simulink model "motor_control"  (Simulink 7.9)
settings: Solver=ode45  StartTime=0.0  StopTime=1  RelTol=1e-3
libraries: powerlib x10
settings Model: Creator=Dmitriy  LastModifiedBy=Dmitriy
settings GRTTargetCC: CombineOutputUpdateFcns=off  GRTInterface=on

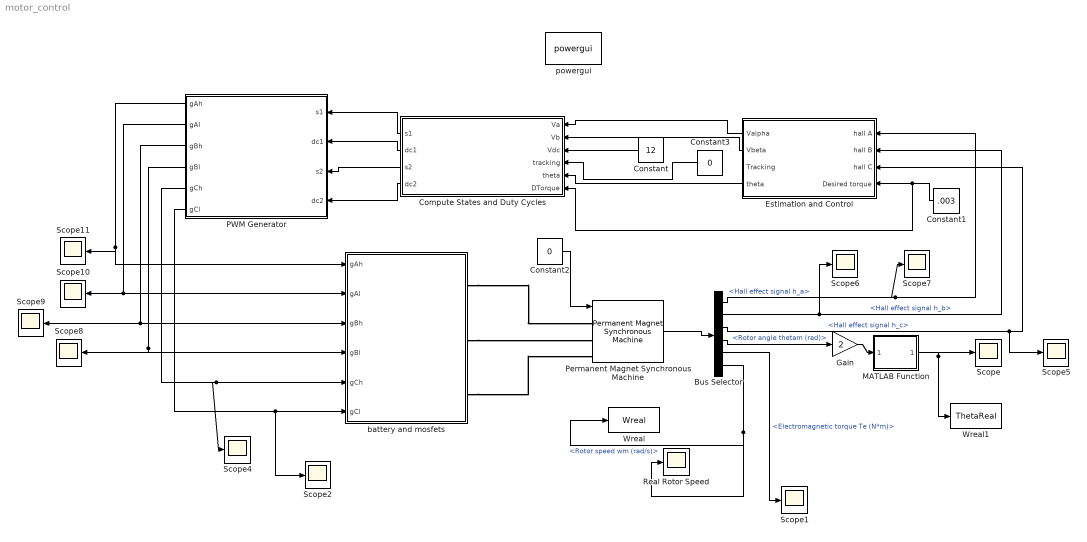
== system motor_control ==
  Bus Selector : BusSelector  OutputSignals=Hall effect signal h_a,Hall effect signal h_b,Hall effect signal h_c,Rotor angle thetam (rad),Electromagnetic torque Te (N*m),Rotor speed wm (rad/s)
  Compute States and Duty Cycles : MATLAB Function  TreatAsAtomicUnit=on  SystemSampleTime=.001
  Constant : Constant  Value=12
  Constant1 : Constant  Value=.003
  Constant2 : Constant  Value=0
  Constant3 : Constant  Value=0
  Estimation and Control : Subsystem  SystemSampleTime=.001
  Gain : Gain  Gain=2
  MATLAB Function : MATLAB Function  TreatAsAtomicUnit=on
  PWM Generator : MATLAB Function  TreatAsAtomicUnit=on  SystemSampleTime=10^-6
  Permanent Magnet Synchronous Machine : powerlib/Machines/Permanent Magnet Synchronous Machine  NbPhases=3  FluxDistribution=Sinusoidal  RotorType=Round  MechanicalLoad=Torque Tm  PresetModel=No  ShowDetailedParameters=on  Resistance=28.2  Inductance=8.5e-3  dqInductances=[0.006365 0.006365]  La=1940*10^-6  MachineConstant=Torque Constant (N.m / A_peak)  Flux=0.0060333  VoltageCst=2.1887  TorqueCst=0.0181  Flat=120  Mechanical=[0.0001 5.396e-005 2 0]  PolePairs=2  InitialConditions=[0,1, 0,0]  InitialConditions5ph=[0 0 0 0 0 0]  TsPowergui=0  TsBlock=-1  RefAngle=Aligned with phase A axis (original Park)
  Real Rotor Speed : Scope
      settings: SaveName=ScopeData18
  Scope{,1..2,4..11} (11 alike) : Scope
      Scope settings: YMin=0.2591  YMax=0.2614
      Scope10 settings: SaveName=ScopeData10
      Scope11 settings: SaveName=ScopeData11
      Scope2 settings: YMin=0.95  YMax=1.05  SaveName=ScopeData2
      Scope4 settings: YMin=0.95  YMax=1.05  SaveName=ScopeData4
      Scope5 settings: SaveName=ScopeData5
      Scope6 settings: SaveName=ScopeData6
      Scope7 settings: SaveName=ScopeData7
      Scope8 settings: SaveName=ScopeData8
      Scope9 settings: SaveName=ScopeData9
  Wreal : ToWorkspace  VariableName=Wreal  SampleTime=-1  SaveFormat=Timeseries
  Wreal1 : ToWorkspace  VariableName=ThetaReal  SampleTime=-1  SaveFormat=Timeseries
  battery and mosfets : Subsystem
  powergui : powerlib/powergui  Priority=1  SimulationMode=Continuous  SolverType=Tustin  SampleTime=50e-6  frequency=60  SPID=off  DisableSnubberDevices=off  DisableRonSwitches=off  DisableVfSwitches=off  SwTol=0  Interpol=off  DisplayEquations=off  FunctionMessages=off  frequencyindice=0  Pbase=100e6  ErrMax=1e-4  Iterations=50  UnitsV=kV  UnitsW=MW  echomessages=off  HookPort=off  EnableUseOfTLC=off  x0status=blocks  RestoreLinks=warning  ResistiveCurrentMeasurement=off  Ylog=off  Xlog=on  ShowGrid=off  save=off  variable=ZData  ZoomFFT=off  StartTime=0.0  cycles=1  DisplayStyle=1  FreqAxis=off  MaxFrequency=1000  frequencyindicesteady=1  display=off  methode=off
  wires:
  Permanent Magnet Synchronous Machine/1 -> Bus Selector/1
  Bus Selector/1 -> Estimation and Control/1(hall A), Scope7/1  "<Hall effect signal h_a>"
  Bus Selector/3 -> Estimation and Control/3(hall C), Scope5/1  "<Hall effect signal h_c>"
  Bus Selector/4 -> Gain/1  "<Rotor angle thetam (rad)>"
  Bus Selector/5 -> Scope1/1  "<Electromagnetic torque Te (N*m)>"
  Bus Selector/2 -> Estimation and Control/2(hall B), Scope6/1  "<Hall effect signal h_b>"
  Estimation and Control/1(Valpha) -> Compute States and Duty Cycles/1(Va)
  Compute States and Duty Cycles/1(s1) -> PWM Generator/1(s1)
  Compute States and Duty Cycles/2(dc1) -> PWM Generator/2(dc1)
  Compute States and Duty Cycles/3(s2) -> PWM Generator/3(s2)
  Compute States and Duty Cycles/4(dc2) -> PWM Generator/4(dc2)
  PWM Generator/6(gCl) -> battery and mosfets/6(gCl), Scope2/1
  PWM Generator/5(gCh) -> battery and mosfets/5(gCh), Scope4/1
  PWM Generator/4(gBl) -> battery and mosfets/4(gBl), Scope8/1
  PWM Generator/3(gBh) -> battery and mosfets/3(gBh), Scope9/1
  PWM Generator/2(gAl) -> battery and mosfets/2(gAl), Scope10/1
  PWM Generator/1(gAh) -> battery and mosfets/1(gAh), Scope11/1
  Constant/1 -> Compute States and Duty Cycles/3(Vdc)
  Constant1/1 -> Estimation and Control/4(Desired torque), Compute States and Duty Cycles/6(DTorque)
  Estimation and Control/2(Vbeta) -> Compute States and Duty Cycles/2(Vb)
  Bus Selector/6 -> Real Rotor Speed/1, Wreal/1  "<Rotor speed wm (rad/s)>"
  MATLAB Function/1(lambda1) -> Wreal1/1, Scope/1
  Gain/1 -> MATLAB Function/1(lambda)
  Constant2/1 -> Permanent Magnet Synchronous Machine/1
  Estimation and Control/4(theta) -> Compute States and Duty Cycles/5(theta)
  Constant3/1 -> Compute States and Duty Cycles/4(tracking)
  connections:
  battery and mosfets/RConn1 -- Permanent Magnet Synchronous Machine/LConn1
  battery and mosfets/RConn2 -- Permanent Magnet Synchronous Machine/LConn2
  battery and mosfets/RConn3 -- Permanent Magnet Synchronous Machine/LConn3

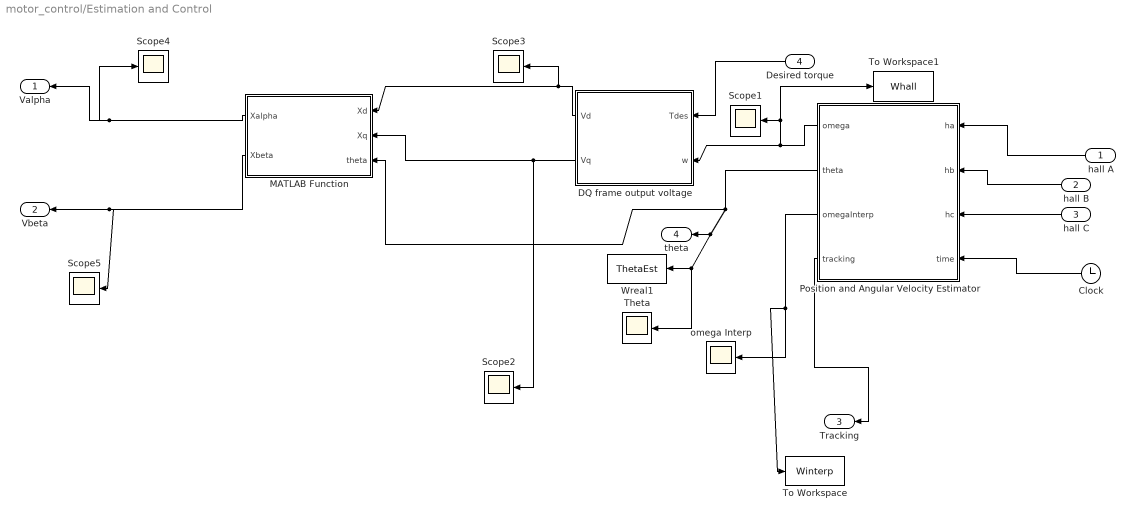
== system motor_control/Estimation and Control ==
  hall A : Inport
  hall B : Inport  Port=2
  hall C : Inport  Port=3
  Desired torque : Inport  Port=4
  Clock : Clock
  DQ frame output voltage : MATLAB Function  TreatAsAtomicUnit=on  SystemSampleTime=.0001
  MATLAB Function : MATLAB Function  TreatAsAtomicUnit=on
  Position and Angular Velocity Estimator : MATLAB Function  TreatAsAtomicUnit=on  SystemSampleTime=.0001
  Scope{1..5} (5 alike) : Scope
      Scope1 settings: SaveName=ScopeData13
      Scope2 settings: SaveName=ScopeData14
      Scope3 settings: SaveName=ScopeData15
      Scope4 settings: SaveName=ScopeData16
      Scope5 settings: SaveName=ScopeData17
  Theta : Scope
      settings: YMin=0  YMax=3.25  SaveName=ScopeData12
  To Workspace : ToWorkspace  VariableName=Winterp  SampleTime=-1  SaveFormat=Timeseries
  To Workspace1 : ToWorkspace  VariableName=Whall  SampleTime=-1  SaveFormat=Timeseries
  Wreal1 : ToWorkspace  VariableName=ThetaEst  SampleTime=-1  SaveFormat=Timeseries
  omega Interp : Scope
      settings: YMin=0  YMax=3.25  SaveName=ScopeData19
  Valpha : Outport
  Vbeta : Outport  Port=2
  Tracking : Outport  Port=3
  theta : Outport  Port=4
  wires:
  Position and Angular Velocity Estimator/1(omega) -> DQ frame output voltage/2(w), Scope1/1, To Workspace1/1
  Desired torque/1 -> DQ frame output voltage/1(Tdes)
  hall A/1 -> Position and Angular Velocity Estimator/1(ha)
  hall B/1 -> Position and Angular Velocity Estimator/2(hb)
  hall C/1 -> Position and Angular Velocity Estimator/3(hc)
  Position and Angular Velocity Estimator/2(theta) -> MATLAB Function/3(theta), Theta/1, Wreal1/1, theta/1
  DQ frame output voltage/2(Vq) -> Scope2/1, MATLAB Function/2(Xq)
  DQ frame output voltage/1(Vd) -> Scope3/1, MATLAB Function/1(Xd)
  MATLAB Function/1(Xalpha) -> Valpha/1, Scope4/1
  MATLAB Function/2(Xbeta) -> Vbeta/1, Scope5/1
  Position and Angular Velocity Estimator/3(omegaInterp) -> omega Interp/1, To Workspace/1
  Clock/1 -> Position and Angular Velocity Estimator/4(time)
  Position and Angular Velocity Estimator/4(tracking) -> Tracking/1

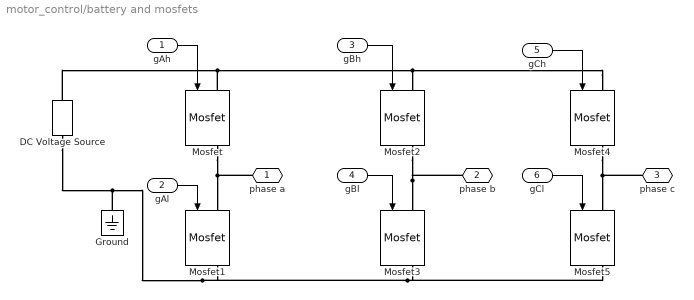
== system motor_control/battery and mosfets ==
  gAh : Inport
  gAl : Inport  Port=2
  gBh : Inport  Port=3
  gBl : Inport  Port=4
  gCh : Inport  Port=5
  gCl : Inport  Port=6
  DC Voltage Source : powerlib/Electrical Sources/DC Voltage Source  Amplitude=12  Measurements=None
  Ground : powerlib/Elements/Ground  LConnTagsString=a
  Mosfet{,1..5} (6 alike) : powerlib/Power Electronics/Mosfet  Ron=0.1  Lon=0  Rd=0.01  Vfd=0  IC=0  Rs=1e5  Cs=inf  Measurements=on
  phase a : PMIOPort  Port=1  Side=Right
  phase b : PMIOPort  Port=2  Side=Right
  phase c : PMIOPort  Port=3  Side=Right
  wires:
  gCl/1 -> Mosfet5/1
  gCh/1 -> Mosfet4/1
  gBh/1 -> Mosfet2/1
  gBl/1 -> Mosfet3/1
  gAl/1 -> Mosfet1/1
  gAh/1 -> Mosfet/1
  connections:
  Mosfet/RConn1 -- Mosfet1/LConn1 -- phase a/RConn1
  Mosfet2/RConn1 -- Mosfet3/LConn1 -- phase b/RConn1
  phase c/RConn1 -- Mosfet4/RConn1 -- Mosfet5/LConn1
  Mosfet1/RConn1 -- Ground/LConn1 -- DC Voltage Source/LConn1 -- Mosfet3/RConn1 -- Mosfet5/RConn1
  Mosfet4/LConn1 -- Mosfet/LConn1 -- DC Voltage Source/RConn1 -- Mosfet2/LConn1

== matlab function Estimation and Control/DQ frame output voltage ==
  data: Tdes input double; Vd output double; w input double; Vq output double
function [Vd,Vq] = computeDQOutput(Tdes,w)
%#codegen
%take the desired torque current 
% speed and compute the output voltage vector in the DQ
%frame. 

L = 1940*10^-6;
R = 28.2;
Ke = (1.895*10^-3)*9.54929659643; % convert to V/(rad/s) 
Kt = 1.81*10^3; %Nm/Amp

%because I is assumed to be on Q axis, T = KtI
Ides = Tdes/Kt;

%bemf is on q axis
bemf = Ke*w;

%inductor impedance 
ZL = L*w;

Vq = bemf+Ides*R;
Vd = -ZL*Ides;

== matlab function Estimation and Control/Position and Angular Velocity Estimator ==
  data: omega output double; ha input double; theta output double; hb input double; hc input double; omegaInterp output double; time input double; tracking output double
function [omega,theta, omegaInterp, tracking] = rotor_est(ha,hb,hc,time)
%#codegen

%estimate the position of the rotor in degrees electrical
%tracking is 0 or 1, 0 means the estimate is bad. Used for activating block
%commutation at initialization
omega=0;
theta=0;
omegaInterp = 0;
time
tracking =0;
coder.extrinsic('rotor_estimate');

[omega theta omegaInterp tracking] = rotor_estimate(ha,hb,hc,time);
end

== matlab function Compute States and Duty Cycles ==
  data: Va input double; s1 output double; dc1 output double; Vb input double; s2 output double; Vdc input double; dc2 output double; tracking input double; theta input double; DTorque input double
function [s1,dc1, s2, dc2] = statesAndCycles(Va,Vb, Vdc, tracking, theta, DTorque)
%#codegen

if(tracking == 1)
    %Given desired Valpha and Vbeta, and the supply voltage, compute the inverter states to toggle
    %between and the duty cycle of each
    
    %right now we're saying that the length of each state vector is Vdc, which
    %is probably wrong
    
    ang = wrapTo2Pi(angle(Va+1i*Vb));
    
    sext = floor(ang/(pi/3));
    
    v1 = 1 +1i;
    v2 = 1 + 1i;
    
    %states as defined in james mevey's thesis
    %v1, v2 are complex values of the voltages
    switch sext
        case 0
            s1 = 1;
            v1 = Vdc;
            
            s2 = 2;
            [t1 t2] = pol2cart(Vdc, pi/3);
            v2 = t1+1i*t2;
            
        case 1
            s1 = 2;
            [t1 t2] = pol2cart(Vdc, pi/3);
            v1 = t1+1i*t2;
            
            s2 = 3;
            [t1 t2] = pol2cart(Vdc, 2*pi/3);
            v2 = t1+1i*t2;
            
        case 2
            s1 = 3;
            [t1 t2] = pol2cart(Vdc, 2*pi/3);
            v1 = t1+1i*t2;
            
            s2 = 4;
            [t1 t2] = pol2cart(Vdc, pi);
            v2 = t1+1i*t2;
        case 3
            s1 = 4;
            [t1 t2] = pol2cart(Vdc, pi);
            v1 = t1+1i*t2;
            
            s2 = 5;
            [t1 t2] = pol2cart(Vdc, 4*pi/3);
            v2 = t1+1i*t2;
        case 4
            s1 = 5;
            [t1 t2] = pol2cart(Vdc, 4*pi/3);
            v1 = t1+1i*t2;
            
            
            s2 = 6;
            [t1 t2] = pol2cart(Vdc, 5*pi/3);
            v2 = t1+1i*t2;
        case 5
            s1 = 6;
            [t1 t2] = pol2cart(Vdc, 5*pi/3);
            v1 = t1+1i*t2;
            
            s2 = 1;
            v2 = Vdc;
        otherwise
            s1 = 0;
            s2 = 0;
    end
    
    %solve for intersection of v1 line and v2 line translated to the desired
    %place
    
    num = Va-imag(v2)*Vb/real(v2)- imag(v1);
    den = real(v1) - imag(v2)/real(v2);
    
    xint = num/den;
    yint = (imag(v1)/real(v1))*xint;
    
    %duty cycle 1 equals length of sv1 divided by Vdc, which is nominal length
    dc1 = sqrt(xint^2+yint^2)/Vdc;
    
    %duty cycle 2 is distance from the tip of sv1 to the desired point, divided
    %by Vdc
    
    dc2 = sqrt((xint-Va)^2 +(yint - Vb)^2)/Vdc;
    
else
    %if not tracking, just use block commutation. The duty cycle is the
    %length of the voltage vector divided by Vdc
    s2 = 0;
    dc2 = 0;
    ang = floor(theta/6);
    dc1 = sqrt(Va^2+Vb^2)/Vdc;
    
    switch(ang)
        case 0
            if(DTorque >= 0)
                s1 = 2;
            else
                s1 = 6;
            end
            
        case 1
            if(DTorque >= 0)
                s1 = 3;
            else
                s1 = 1;
            end
            
        case 2
            if(DTorque >= 0)
                s1 = 4;
            else
                s1 = 2;
            end
        case 3
            if(DTorque >= 0)
                s1 = 5;
            else
                s1 = 3;
            end
        case 4
            if(DTorque >= 0)
                s1 = 6;
            else
                s1 = 4;
            end
        case 5
            if(DTorque >= 0)
                s1 = 1;
            else
                s1 = 5;
            end
        otherwise
            s1=0;
    end
end



end

function lambda = wrapTo2Pi(lambda)
%wrapTo2Pi Wrap angle in radians to [0 2*pi]
%
%   lambdaWrapped = wrapTo2Pi(LAMBDA) wraps angles in LAMBDA, in radians,
%   to the interval [0 2*pi] such that zero maps to zero and 2*pi maps
%   to 2*pi. (In general, positive multiples of 2*pi map to 2*pi and
%   negative multiples of 2*pi map to zero.)
%
%   See also wrapToPi, wrapTo180, wrapTo360.

% Copyright 2007-2008 The MathWorks, Inc.
% $Revision: 1.1.6.1 $  $Date: 2008/12/22 23:50:53 $

positiveInput = (lambda > 0);
lambda = mod(lambda, 2*pi);
lambda((lambda == 0) & positiveInput) = 2*pi;
end

function p = angle(h)
%ANGLE  Phase angle.
%   ANGLE(H) returns the phase angles, in radians, of a matrix with
%   complex elements.
%
%   Class support for input X:
%      float: double, single
%
%   See also ABS, UNWRAP.

%   Copyright 1984-2010 The MathWorks, Inc.
%   $Revision: 5.7.4.2 $  $Date: 2010/04/21 21:31:19 $

p = atan2(imag(h), real(h));
end

== matlab function PWM Generator ==
  data: s1 input double; gAh output double; dc1 input double; s2 input double; dc2 input double; gAl output double; gBh output double; gBl output double; gCh output double; gCl output double
function [gAh,gAl,gBh,gBl,gCh,gCl] = generateGateSignals(s1,dc1,s2,dc2)
%#codegen
Tsamp = 10^-6;
Tswitch = 10^-4;



persistent k;

if(isempty(k))
    k=1;
end

if(k > 100)
    k=1;
end

%determine the current output
if(k<100*dc1)
    output = s1;
else
    if(k>100-100*dc2)
        output = s2;
    else
        output = 0;
    end
end

%generate the gate signals
switch output
    case 0
        gates = [0 1 0 1 0 1];
        
    case 1
        gates = [1 0 0 1 0 1];
        
    case 2
        gates = [1 0 1 0 0 1];
        
    case 3
        gates = [0 1 1 0 0 1];
        
    case 4
        gates = [0 1 1 0 1 0];
        
    case 5
        gates = [0 1 0 1 0 0];
    
    case 6
        gates = [1 0 0 1 1 0];
        
    otherwise
        gates = [ 0 0 0 0 0 0];
end

%only for testing other parts of the sim
%gates= [ 0 0 0 0 0 0];

gAh = gates(1);
gAl = gates(2);
gBh = gates(3);
gBl = gates(4);
gCh = gates(5);
gCl = gates(6);

% k=k+1;

== matlab function MATLAB Function ==
  data: lambda input double; lambda1 output double
function lambda1 = wrapTo2Pi(lambda)
%wrapTo2Pi Wrap angle in radians to [0 2*pi]
%
%   lambdaWrapped = wrapTo2Pi(LAMBDA) wraps angles in LAMBDA, in radians,
%   to the interval [0 2*pi] such that zero maps to zero and 2*pi maps
%   to 2*pi. (In general, positive multiples of 2*pi map to 2*pi and
%   negative multiples of 2*pi map to zero.)
%
%   See also wrapToPi, wrapTo180, wrapTo360.

% Copyright 2007-2008 The MathWorks, Inc.
% $Revision: 1.1.6.1 $  $Date: 2008/12/22 23:50:53 $


positiveInput = (lambda > 0);
lambda = mod(lambda, 2*pi);
lambda((lambda == 0) & positiveInput) = 2*pi;
lambda1=lambda;
end

== matlab function Estimation and Control/MATLAB Function ==
  data: Xd input double; Xalpha output double; Xq input double; theta input double; Xbeta output double
function [Xalpha,Xbeta] = inversePark(Xd,Xq,theta)
%#codegen
%implements inverse park as described in james mevey's thesis

c = cos(theta);
s = sin(theta);

ipm = [c -s; s c];

xab = ipm*[Xd Xq]';

Xalpha = xab(1);
Xbeta = xab(2);
end
